simulink model "RoboBoat_NEDcallv12"  (R2014a)
settings: Solver=FixedStepDiscrete  StartTime=0.0  StopTime=inf  FixedStep=.1  RelTol=1e-3
undefined symbols (not defined in the file): Com1, Com2, Com3, Com4, DiscIntNeverNeededParam, standard
libraries: xpcseriallib x31, visiontextngfix x25, simulink x19, slrtlib x9, speedgoatlib_IO102 x3, speedgoatlib x1
(part 4 of 4)

== matlab function RoboBoat_NEDcallv12/Main FSM/Obstacle Navigation1/Exit Gate/Gate 1 (Red & White)/MATLAB Function ==
  data: Prob input; RPM output; ColorID input; Dist input; Ang input; CurrentHeading input; GPSLat input; GPSLong input; Timer input; DesiredHeading output; gateGPS output
function [RPM,DesiredHeading,gateGPS] = navigation(Prob,ColorID,Dist,Ang,CurrentHeading,GPSLat,GPSLong,Timer)

% Function performs one buoy navigation through the start speed gates. If
% no buoys are found by the LIDAR/Vision assembly then an incremented
% turning algorithm is executed to turn by 10 degrees per increment up to 
% 90 degrees either way of the inital heading

% Written by Edward Zhu

persistent LockHeading TimeLastFound Counter Turn TurnInc gateLat gateLong

if isempty(LockHeading) && isempty(TimeLastFound) && isempty(Counter) && isempty(Turn) && isempty(TurnInc)
    LockHeading = CurrentHeading;
    TimeLastFound = 0;
    Counter = 0;
    TurnInc = 30;
    Turn = TurnInc;
    gateLat = 0;
    gateLong = 0;
end

Distance = Dist/100;

BoatWidth = 0.75;
Buffer = atan(2*BoatWidth/Distance);

RedOffset = Ang + Buffer;
WhiteOffset = Ang - Buffer;

R = 6378137;

CurLat = (floor(GPSLat/100)+mod(GPSLat,100)/60)*pi/180;
CurLong = (ceil(GPSLong/100)-mod(-GPSLong,100)/60)*pi/180;

gateHeading = (mod(CurrentHeading + Ang, 360))*pi/180;

if ColorID == 1 && Prob > 0.9
    if Ang < 0
        DesiredHeading = mod(CurrentHeading - RedOffset, 360);
    else
        DesiredHeading = mod(CurrentHeading + RedOffset, 360);
    end
    RPM = 4000;
    GateFound = 1;
    TimeLastFound = Timer;
    gateLat =  asin(sin(CurLat)*cos(Distance/R) + cos(CurLat)*sin(Distance/R)*cos(gateHeading))*180/pi;
    gateLong = (CurLong + atan2(sin(gateHeading)*sin(Distance/R)*cos(CurLat),cos(Distance/R)-sin(CurLat)*sin(gateLat)))*180/pi;
elseif ColorID == 2 && Prob > 0.9
    DesiredHeading = mod(LockHeading - Turn, 360);
    RPM = 0;
    GateFound = 1;
    TimeLastFound = Timer;
%     DesiredHeading = mod(CurrentHeading - WhiteOffset, 360);
%     RPM = 4000;
%     GateFound = 1;
%     TimeLastFound = Timer;
%     gateLat =  asin(sin(CurLat)*cos(Distance/R) + cos(CurLat)*sin(Distance/R)*cos(gateHeading))*180/pi;
%     gateLong = (CurLong + atan2(sin(gateHeading)*sin(Distance/R)*cos(CurLat),cos(Distance/R)-sin(CurLat)*sin(gateLat)))*180/pi;
else
    DesiredHeading = CurrentHeading;
    RPM = 0;
    GateFound = 0;
end

gateGPS = [gateLat gateLong];
TimeNoBuoys = Timer - TimeLastFound;

if GateFound == 0 && TimeNoBuoys > 15
    RPM = 0;
    DesiredHeading = mod(LockHeading - Turn, 360);
    HeadingDiff = DesiredHeading - CurrentHeading;
    gateGPS = [gateLat gateLong];
    
    if HeadingDiff > 180
        HeadingDiff = HeadingDiff - 360;
    elseif HeadingDiff < -180
        HeadingDiff = HeadingDiff + 360;
    end
    
    if HeadingDiff < 3
        Counter = Counter + 1;
    else
        Counter = 0;
    end
    
    if Counter >= 15
        Turn = Turn + TurnInc;
        Counter = 0;
        if abs(Turn) > 90
            TurnInc = -TurnInc;
        end
    end
end

== matlab function RoboBoat_NEDcallv12/Main FSM/Obstacle Navigation1/Exit Gate/Gate 2 (White & White)/Distance ==
  data: Distance output; DesiredGPS input; GPSLat input; GPSLong input
function Distance  = DistCalc(DesiredGPS, GPSLat, GPSLong)

%Written by Anderson Lebbad on July 22, 2013
%Last Edited:

%Orients the boat towards a target GPS point before approaching it.
%This is done to keep the approach angle minimal, so the approach
%algorithm does not circle the target and never reach it.

%Parse input GPS and convert angles to radians
CurLat = (floor(GPSLat/100)+mod(GPSLat,100)/60)*pi/180;
CurLong = (floor(GPSLong/100)+mod(GPSLong,100)/60)*pi/180;
DesLat = (floor(DesiredGPS(1)/100)+mod(DesiredGPS(1),100)/60)*pi/180;
DesLong = (floor(DesiredGPS(2)/100)+mod(DesiredGPS(2),100)/60)*pi/180;
%Difference between lats and longs
DiffLat = DesLat - CurLat;
MidLat = cos((CurLat + DesLat)/2);
DiffLong = DesLong - CurLong;
%Radius of the earth in meters
R = 6378137;

%Calculate distance using the great-circle distance formula
%Formula documented here:
%   http://www.movable-type.co.uk/scripts/latlong.html
% a = sin(DiffLat/2)^2+sin(DiffLong/2)^2*cos(CurLat)*cos(DesLat);
% c = 2*atan2(sqrt(a), sqrt(1-a));
% Distance = R*c;

%Calculating distance using Pythagora's
a = DiffLong*MidLat;
b = DiffLat;
Distance = R*sqrt(a^2+b^2);

== matlab function RoboBoat_NEDcallv12/Sensors/Baseboard Serial/GPS Decode/LLA to NED ==
  data: GPSLat input; GPSLong input; Lat output; Long output
function [Lat, Long] = LLA2NEDfun(GPSLat,GPSLong)
%Written by Anderson Lebbad on September 20, 2014
%Last edited by:
%
%This function converts the NMEA formatted GPS values to degrees for
%latitude and longitude.

Lat = (floor(GPSLat/100)+mod(GPSLat,100)/60);
%Negative added for being in western hemisphere
Long = -(ceil(GPSLong/100)-mod(-GPSLong,100)/60);

end

== matlab function RoboBoat_NEDcallv12/Main FSM/Obstacle Navigation1/Exit Gate/Gate 2 (White & White)/MATLAB Function ==
  data: Prob input; RPM output; ColorID input; Dist input; Ang input; CurrentHeading input; GPSLat input; GPSLong input; Timer input; DesiredHeading output; gateGPS output
function [RPM,DesiredHeading,gateGPS] = navigation(Prob,ColorID,Dist,Ang,CurrentHeading,GPSLat,GPSLong,Timer)

% Function performs one buoy navigation through the start speed gates. If
% no buoys are found by the LIDAR/Vision assembly then an incremented
% turning algorithm is executed to turn by 10 degrees per increment up to 
% 90 degrees either way of the inital heading

% Written by Edward Zhu


persistent LockHeading TimeLastFound Counter Turn TurnInc gateLat gateLong

if isempty(LockHeading) && isempty(TimeLastFound) && isempty(Counter) && isempty(Turn) && isempty(TurnInc)
    LockHeading = CurrentHeading;
    TimeLastFound = 0;
    Counter = 0;
    TurnInc = 30;
    Turn = TurnInc;
    gateLat = 0;
    gateLong = 0;
end
Distance = Dist/100;
BoatWidth = 0.75;
Buffer = atan(2*BoatWidth/Distance);

RedOffset = Ang + Buffer;
WhiteOffset = Ang - Buffer;

R = 6378137;

CurLat = (floor(GPSLat/100)+mod(GPSLat,100)/60)*pi/180;
CurLong = (ceil(GPSLong/100)-mod(-GPSLong,100)/60)*pi/180;

gateHeading = (mod(CurrentHeading - Ang, 360))*pi/180;

if ColorID == 1 && Prob > 0.9
    DesiredHeading = mod(CurrentHeading - RedOffset, 360);
    RPM = 2000;
    GateFound = 1;
    TimeLastFound = Timer;
    gateLat =  asin(sin(CurLat)*cos(Distance/R) + cos(CurLat)*sin(Distance/R)*cos(gateHeading))*180/pi;
    gateLong = (CurLong + atan2(sin(gateHeading)*sin(Distance/R)*cos(CurLat),cos(Distance/R)-sin(CurLat)*sin(gateLat)))*180/pi;
elseif ColorID == 2 && Prob > 0.9
    DesiredHeading = mod(CurrentHeading - WhiteOffset, 360);
    RPM = 2000;
    GateFound = 1;
    TimeLastFound = Timer;
    gateLat =  asin(sin(CurLat)*cos(Distance/R) + cos(CurLat)*sin(Distance/R)*cos(gateHeading))*180/pi;
    gateLong = (CurLong + atan2(sin(gateHeading)*sin(Distance/R)*cos(CurLat),cos(Distance/R)-sin(CurLat)*sin(gateLat)))*180/pi;
else
    DesiredHeading = CurrentHeading;
    RPM = 0;
    GateFound = 0;
end

gateGPS = [gateLat gateLong];
TimeNoBuoys = Timer - TimeLastFound;

if GateFound == 0 && TimeNoBuoys > 15
    RPM = 0;
    DesiredHeading = mod(LockHeading - Turn, 360);
    HeadingDiff = DesiredHeading - CurrentHeading;
    gateGPS = [gateLat gateLong];
    
    if HeadingDiff > 180
        HeadingDiff = HeadingDiff - 360;
    elseif HeadingDiff < -180
        HeadingDiff = HeadingDiff + 360;
    end
    
    if HeadingDiff < 3
        Counter = Counter + 1;
    else
        Counter = 0;
    end
    
    if Counter >= 15
        Turn = Turn + TurnInc;
        Counter = 0;
        if abs(Turn) > 90
            TurnInc = -TurnInc;
        end
    end
end

== matlab function RoboBoat_NEDcallv12/Main FSM/Obstacle Navigation1/Exit Gate/Gate 3 (White & Green)/Distance ==
  data: Distance output; DesiredGPS input; GPSLat input; GPSLong input
function Distance  = DistCalc(DesiredGPS, GPSLat, GPSLong)

%Written by Anderson Lebbad on July 22, 2013
%Last Edited:

%Orients the boat towards a target GPS point before approaching it.
%This is done to keep the approach angle minimal, so the approach
%algorithm does not circle the target and never reach it.

%Parse input GPS and convert angles to radians
CurLat = (floor(GPSLat/100)+mod(GPSLat,100)/60)*pi/180;
CurLong = (floor(GPSLong/100)+mod(GPSLong,100)/60)*pi/180;
DesLat = (floor(DesiredGPS(1)/100)+mod(DesiredGPS(1),100)/60)*pi/180;
DesLong = (floor(DesiredGPS(2)/100)+mod(DesiredGPS(2),100)/60)*pi/180;
%Difference between lats and longs
DiffLat = DesLat - CurLat;
MidLat = cos((CurLat + DesLat)/2);
DiffLong = DesLong - CurLong;
%Radius of the earth in meters
R = 6378137;

%Calculate distance using the great-circle distance formula
%Formula documented here:
%   http://www.movable-type.co.uk/scripts/latlong.html
% a = sin(DiffLat/2)^2+sin(DiffLong/2)^2*cos(CurLat)*cos(DesLat);
% c = 2*atan2(sqrt(a), sqrt(1-a));
% Distance = R*c;

%Calculating distance using Pythagora's
a = DiffLong*MidLat;
b = DiffLat;
Distance = R*sqrt(a^2+b^2);

== matlab function RoboBoat_NEDcallv12/Main FSM/Obstacle Navigation1/Exit Gate/Gate 3 (White & Green)/MATLAB Function ==
  data: Prob input; RPM output; ColorID input; Dist input; Ang input; CurrentHeading input; GPSLat input; GPSLong input; Timer input; DesiredHeading output; gateGPS output
function [RPM,DesiredHeading,gateGPS] = navigation(Prob,ColorID,Dist,Ang,CurrentHeading,GPSLat,GPSLong,Timer)

% Function performs one buoy navigation through the start speed gates. If
% no buoys are found by the LIDAR/Vision assembly then an incremented
% turning algorithm is executed to turn by 10 degrees per increment up to 
% 90 degrees either way of the inital heading

% Written by Edward Zhu


persistent LockHeading TimeLastFound Counter Turn TurnInc gateLat gateLong

if isempty(LockHeading) && isempty(TimeLastFound) && isempty(Counter) && isempty(Turn) && isempty(TurnInc)
    LockHeading = CurrentHeading;
    TimeLastFound = 0;
    Counter = 0;
    TurnInc = 30;
    Turn = TurnInc;
    gateLat = 0;
    gateLong = 0;
end
Distance = Dist/100;
BoatWidth = 0.75;
Buffer = atan(2*BoatWidth/Distance);

WhiteOffset = Ang + Buffer;
GreenOffset = Ang - Buffer;

R = 6378137;

CurLat = (floor(GPSLat/100)+mod(GPSLat,100)/60)*pi/180;
CurLong = (ceil(GPSLong/100)-mod(-GPSLong,100)/60)*pi/180;

gateHeading = (mod(CurrentHeading - Ang, 360))*pi/180;

if ColorID == 2 && Prob > 0.9
    DesiredHeading = mod(LockHeading - Turn, 360);
    RPM = 0;
    GateFound = 1;
    TimeLastFound = Timer;
elseif ColorID == 3 && Prob > 0.9
    if Ang > 0
        DesiredHeading = mod(CurrentHeading - GreenOffset, 360);
    else
        DesiredHeading = mod(CurrentHeading + GreenOffset, 360);
    end
    RPM = 4000;
    GateFound = 1;
    TimeLastFound = Timer;
    gateLat =  asin(sin(CurLat)*cos(Distance/R) + cos(CurLat)*sin(Distance/R)*cos(gateHeading))*180/pi;
    gateLong = (CurLong + atan2(sin(gateHeading)*sin(Distance/R)*cos(CurLat),cos(Distance/R)-sin(CurLat)*sin(gateLat)))*180/pi;
else
    DesiredHeading = CurrentHeading;
    RPM = 0;
    GateFound = 0;
end

gateGPS = [gateLat gateLong];
TimeNoBuoys = Timer - TimeLastFound;

if GateFound == 0 && TimeNoBuoys > 15
    RPM = 0;
    DesiredHeading = mod(LockHeading - Turn, 360);
    HeadingDiff = DesiredHeading - CurrentHeading;
    gateGPS = [gateLat gateLong];
    
    if HeadingDiff > 180
        HeadingDiff = HeadingDiff - 360;
    elseif HeadingDiff < -180
        HeadingDiff = HeadingDiff + 360;
    end
    
    if HeadingDiff < 3
        Counter = Counter + 1;
    else
        Counter = 0;
    end
    
    if Counter >= 15
        Turn = Turn + TurnInc;
        Counter = 0;
        if abs(Turn) > 90
            TurnInc = -TurnInc;
        end
    end
end

== matlab function RoboBoat_NEDcallv12/Main FSM/Obstacle Navigation1/Exit Gate/MATLAB Function ==
  data: gateID input; outputSelector output; gate1En output; gate2En output; gate3En output
function [outputSelector,gate1En,gate2En,gate3En] = gateSelector(gateID)
% Determines which colors to filter for based on the gateID as received
% from the judges

gate1En = 0;
gate2En = 0;
gate3En = 0;

if gateID == 1
    gate1En = 1;
    outputSelector = 1;
elseif gateID == 2
    gate2En = 1;
    outputSelector = 2;
else
    gate3En = 1;
    outputSelector = 3;
end

== matlab function RoboBoat_NEDcallv12/Sinks/actuators/analog output/Subsystem/Heading Controller/MATLAB Function ==
  data: HeadingDesired input; steering output; CompassHeading input
function steering = CalcSteering(HeadingDesired, CompassHeading)

%Written by Anderson Lebbad on May 29, 2015
%Last Edited: Anderson Lebbad on June 7, 2015
%   Simplified using mod division

%Calculates the difference between the desired and current heading to be
%used for steering

steering = HeadingDesired - CompassHeading;
%atan2 in radians, input and output in degrees
steering = atan2(sin(steering*pi/180),cos(steering*pi/180))*180/pi;

== matlab function RoboBoat_NEDcallv12/Main FSM/Obstacle Navigation1/Enter Gate/Gate 1 (Red & White)/Distance ==
  data: Distance output; DesiredGPS input; GPSLat input; GPSLong input
function Distance  = DistCalc(DesiredGPS, GPSLat, GPSLong)

%Written by Anderson Lebbad on July 22, 2013
%Last Edited:

%Orients the boat towards a target GPS point before approaching it.
%This is done to keep the approach angle minimal, so the approach
%algorithm does not circle the target and never reach it.

%Parse input GPS and convert angles to radians
CurLat = (floor(GPSLat/100)+mod(GPSLat,100)/60)*pi/180;
CurLong = (floor(GPSLong/100)+mod(GPSLong,100)/60)*pi/180;
DesLat = (floor(DesiredGPS(1)/100)+mod(DesiredGPS(1),100)/60)*pi/180;
DesLong = (floor(DesiredGPS(2)/100)+mod(DesiredGPS(2),100)/60)*pi/180;
%Difference between lats and longs
DiffLat = DesLat - CurLat;
MidLat = cos((CurLat + DesLat)/2);
DiffLong = DesLong - CurLong;
%Radius of the earth in meters
R = 6378137;

%Calculate distance using the great-circle distance formula
%Formula documented here:
%   http://www.movable-type.co.uk/scripts/latlong.html
% a = sin(DiffLat/2)^2+sin(DiffLong/2)^2*cos(CurLat)*cos(DesLat);
% c = 2*atan2(sqrt(a), sqrt(1-a));
% Distance = R*c;

%Calculating distance using Pythagora's
a = DiffLong*MidLat;
b = DiffLat;
Distance = R*sqrt(a^2+b^2);

== matlab function RoboBoat_NEDcallv12/Main FSM/Obstacle Navigation1/Enter Gate/Gate 1 (Red & White)/MATLAB Function ==
  data: Prob input; RPM output; ColorID input; Dist input; Ang input; CurrentHeading input; GPSLat input; GPSLong input; Timer input; DesiredHeading output; gateGPS output
function [RPM,DesiredHeading,gateGPS] = navigation(Prob,ColorID,Dist,Ang,CurrentHeading,GPSLat,GPSLong,Timer)

% Function performs one buoy navigation through the start speed gates. If
% no buoys are found by the LIDAR/Vision assembly then an incremented
% turning algorithm is executed to turn by 10 degrees per increment up to 
% 90 degrees either way of the inital heading

% Written by Edward Zhu

persistent LockHeading TimeLastFound Counter Turn TurnInc gateLat gateLong

if isempty(LockHeading) && isempty(TimeLastFound) && isempty(Counter) && isempty(Turn) && isempty(TurnInc)
    LockHeading = CurrentHeading;
    TimeLastFound = 0;
    Counter = 0;
    TurnInc = 30;
    Turn = TurnInc;
    gateLat = 0;
    gateLong = 0;
end

Distance = Dist/100;

BoatWidth = 0.75;
Buffer = atan(2*BoatWidth/Distance);

RedOffset = Ang + Buffer;
WhiteOffset = Ang - Buffer;

R = 6378137;

CurLat = (floor(GPSLat/100)+mod(GPSLat,100)/60)*pi/180;
CurLong = (ceil(GPSLong/100)-mod(-GPSLong,100)/60)*pi/180;

gateHeading = (mod(CurrentHeading + Ang, 360))*pi/180;

if ColorID == 1 && Prob > 0.9
    if Ang < 0
        DesiredHeading = mod(CurrentHeading - RedOffset, 360);
    else
        DesiredHeading = mod(CurrentHeading + RedOffset, 360);
    end
    RPM = 4000;
    GateFound = 1;
    TimeLastFound = Timer;
    gateLat =  asin(sin(CurLat)*cos(Distance/R) + cos(CurLat)*sin(Distance/R)*cos(gateHeading))*180/pi;
    gateLong = (CurLong + atan2(sin(gateHeading)*sin(Distance/R)*cos(CurLat),cos(Distance/R)-sin(CurLat)*sin(gateLat)))*180/pi;
elseif ColorID == 2 && Prob > 0.9
    DesiredHeading = mod(LockHeading - Turn, 360);
    RPM = 0;
    GateFound = 1;
    TimeLastFound = Timer;
%     DesiredHeading = mod(CurrentHeading - WhiteOffset, 360);
%     RPM = 4000;
%     GateFound = 1;
%     TimeLastFound = Timer;
%     gateLat =  asin(sin(CurLat)*cos(Distance/R) + cos(CurLat)*sin(Distance/R)*cos(gateHeading))*180/pi;
%     gateLong = (CurLong + atan2(sin(gateHeading)*sin(Distance/R)*cos(CurLat),cos(Distance/R)-sin(CurLat)*sin(gateLat)))*180/pi;
else
    DesiredHeading = CurrentHeading;
    RPM = 0;
    GateFound = 0;
end

gateGPS = [gateLat gateLong];
TimeNoBuoys = Timer - TimeLastFound;

if GateFound == 0 && TimeNoBuoys > 15
    RPM = 0;
    DesiredHeading = mod(LockHeading - Turn, 360);
    HeadingDiff = DesiredHeading - CurrentHeading;
    gateGPS = [gateLat gateLong];
    
    if HeadingDiff > 180
        HeadingDiff = HeadingDiff - 360;
    elseif HeadingDiff < -180
        HeadingDiff = HeadingDiff + 360;
    end
    
    if HeadingDiff < 3
        Counter = Counter + 1;
    else
        Counter = 0;
    end
    
    if Counter >= 15
        Turn = Turn + TurnInc;
        Counter = 0;
        if abs(Turn) > 90
            TurnInc = -TurnInc;
        end
    end
end

== matlab function RoboBoat_NEDcallv12/Main FSM/Obstacle Navigation1/Enter Gate/Gate 2 (White & White)/Distance ==
  data: Distance output; DesiredGPS input; GPSLat input; GPSLong input
function Distance  = DistCalc(DesiredGPS, GPSLat, GPSLong)

%Written by Anderson Lebbad on July 22, 2013
%Last Edited:

%Orients the boat towards a target GPS point before approaching it.
%This is done to keep the approach angle minimal, so the approach
%algorithm does not circle the target and never reach it.

%Parse input GPS and convert angles to radians
CurLat = (floor(GPSLat/100)+mod(GPSLat,100)/60)*pi/180;
CurLong = (floor(GPSLong/100)+mod(GPSLong,100)/60)*pi/180;
DesLat = (floor(DesiredGPS(1)/100)+mod(DesiredGPS(1),100)/60)*pi/180;
DesLong = (floor(DesiredGPS(2)/100)+mod(DesiredGPS(2),100)/60)*pi/180;
%Difference between lats and longs
DiffLat = DesLat - CurLat;
MidLat = cos((CurLat + DesLat)/2);
DiffLong = DesLong - CurLong;
%Radius of the earth in meters
R = 6378137;

%Calculate distance using the great-circle distance formula
%Formula documented here:
%   http://www.movable-type.co.uk/scripts/latlong.html
% a = sin(DiffLat/2)^2+sin(DiffLong/2)^2*cos(CurLat)*cos(DesLat);
% c = 2*atan2(sqrt(a), sqrt(1-a));
% Distance = R*c;

%Calculating distance using Pythagora's
a = DiffLong*MidLat;
b = DiffLat;
Distance = R*sqrt(a^2+b^2);

== matlab function RoboBoat_NEDcallv12/Main FSM/Obstacle Navigation1/Enter Gate/Gate 2 (White & White)/MATLAB Function ==
  data: Prob input; RPM output; ColorID input; Dist input; Ang input; CurrentHeading input; GPSLat input; GPSLong input; Timer input; DesiredHeading output; gateGPS output
function [RPM,DesiredHeading,gateGPS] = navigation(Prob,ColorID,Dist,Ang,CurrentHeading,GPSLat,GPSLong,Timer)

% Function performs one buoy navigation through the start speed gates. If
% no buoys are found by the LIDAR/Vision assembly then an incremented
% turning algorithm is executed to turn by 10 degrees per increment up to 
% 90 degrees either way of the inital heading

% Written by Edward Zhu


persistent LockHeading TimeLastFound Counter Turn TurnInc gateLat gateLong

if isempty(LockHeading) && isempty(TimeLastFound) && isempty(Counter) && isempty(Turn) && isempty(TurnInc)
    LockHeading = CurrentHeading;
    TimeLastFound = 0;
    Counter = 0;
    TurnInc = 30;
    Turn = TurnInc;
    gateLat = 0;
    gateLong = 0;
end
Distance = Dist/100;
BoatWidth = 0.75;
Buffer = atan(2*BoatWidth/Distance);

RedOffset = Ang + Buffer;
WhiteOffset = Ang - Buffer;

R = 6378137;

CurLat = (floor(GPSLat/100)+mod(GPSLat,100)/60)*pi/180;
CurLong = (ceil(GPSLong/100)-mod(-GPSLong,100)/60)*pi/180;

gateHeading = (mod(CurrentHeading - Ang, 360))*pi/180;

if ColorID == 1 && Prob > 0.9
    DesiredHeading = mod(CurrentHeading - RedOffset, 360);
    RPM = 2000;
    GateFound = 1;
    TimeLastFound = Timer;
    gateLat =  asin(sin(CurLat)*cos(Distance/R) + cos(CurLat)*sin(Distance/R)*cos(gateHeading))*180/pi;
    gateLong = (CurLong + atan2(sin(gateHeading)*sin(Distance/R)*cos(CurLat),cos(Distance/R)-sin(CurLat)*sin(gateLat)))*180/pi;
elseif ColorID == 2 && Prob > 0.9
    DesiredHeading = mod(CurrentHeading - WhiteOffset, 360);
    RPM = 2000;
    GateFound = 1;
    TimeLastFound = Timer;
    gateLat =  asin(sin(CurLat)*cos(Distance/R) + cos(CurLat)*sin(Distance/R)*cos(gateHeading))*180/pi;
    gateLong = (CurLong + atan2(sin(gateHeading)*sin(Distance/R)*cos(CurLat),cos(Distance/R)-sin(CurLat)*sin(gateLat)))*180/pi;
else
    DesiredHeading = CurrentHeading;
    RPM = 0;
    GateFound = 0;
end

gateGPS = [gateLat gateLong];
TimeNoBuoys = Timer - TimeLastFound;

if GateFound == 0 && TimeNoBuoys > 15
    RPM = 0;
    DesiredHeading = mod(LockHeading - Turn, 360);
    HeadingDiff = DesiredHeading - CurrentHeading;
    gateGPS = [gateLat gateLong];
    
    if HeadingDiff > 180
        HeadingDiff = HeadingDiff - 360;
    elseif HeadingDiff < -180
        HeadingDiff = HeadingDiff + 360;
    end
    
    if HeadingDiff < 3
        Counter = Counter + 1;
    else
        Counter = 0;
    end
    
    if Counter >= 15
        Turn = Turn + TurnInc;
        Counter = 0;
        if abs(Turn) > 90
            TurnInc = -TurnInc;
        end
    end
end

== matlab function RoboBoat_NEDcallv12/Main FSM/Obstacle Navigation1/Enter Gate/Gate 3 (White & Green)/Distance ==
  data: Distance output; DesiredGPS input; GPSLat input; GPSLong input
function Distance  = DistCalc(DesiredGPS, GPSLat, GPSLong)

%Written by Anderson Lebbad on July 22, 2013
%Last Edited:

%Orients the boat towards a target GPS point before approaching it.
%This is done to keep the approach angle minimal, so the approach
%algorithm does not circle the target and never reach it.

%Parse input GPS and convert angles to radians
CurLat = (floor(GPSLat/100)+mod(GPSLat,100)/60)*pi/180;
CurLong = (floor(GPSLong/100)+mod(GPSLong,100)/60)*pi/180;
DesLat = (floor(DesiredGPS(1)/100)+mod(DesiredGPS(1),100)/60)*pi/180;
DesLong = (floor(DesiredGPS(2)/100)+mod(DesiredGPS(2),100)/60)*pi/180;
%Difference between lats and longs
DiffLat = DesLat - CurLat;
MidLat = cos((CurLat + DesLat)/2);
DiffLong = DesLong - CurLong;
%Radius of the earth in meters
R = 6378137;

%Calculate distance using the great-circle distance formula
%Formula documented here:
%   http://www.movable-type.co.uk/scripts/latlong.html
% a = sin(DiffLat/2)^2+sin(DiffLong/2)^2*cos(CurLat)*cos(DesLat);
% c = 2*atan2(sqrt(a), sqrt(1-a));
% Distance = R*c;

%Calculating distance using Pythagora's
a = DiffLong*MidLat;
b = DiffLat;
Distance = R*sqrt(a^2+b^2);

== matlab function RoboBoat_NEDcallv12/Main FSM/Obstacle Navigation1/Obstacle Navigation/GPS: Bee Line/Orient/Desired Heading ==
  data: DesiredGPS input; DesiredHeading output; GPSLat input; GPSLong input
function DesiredHeading = Orient(DesiredGPS, GPSLat, GPSLong)

%Written by Anderson Lebbad on July 22, 2013
%Last Edited: Edward Zhu on July 5, 2014

% Edit:
% Changed calculation to use positive lat and negative long

%Orients the boat towards a target GPS point before approaching it.
%This is done to keep the approach angle minimal, so the approach
%algorithm does not circle the target and never reach it.

%Parse input GPS and convert angles to radians
CurLat = (floor(GPSLat/100)+mod(GPSLat,100)/60)*pi/180;
CurLong = (ceil(GPSLong/100)-mod(-GPSLong,100)/60)*pi/180;
DesLat = (floor(DesiredGPS(1)/100)+mod(DesiredGPS(1),100)/60)*pi/180;
DesLong = (ceil(DesiredGPS(2)/100)-mod(-DesiredGPS(2),100)/60)*pi/180;

%Difference between longs
DiffLong = DesLong - CurLong;

%Calculate initial bearing - formula documented here: 
%   http://www.movable-type.co.uk/scripts/latlong.html
y = sin(DiffLong)*cos(DesLat);
x = cos(CurLat)*sin(DesLat)-sin(CurLat)*cos(DesLat)*cos(DiffLong);
DesiredHeading = mod(atan2(y, x)*180/pi + 360, 360);

== matlab function RoboBoat_NEDcallv12/Main FSM/Obstacle Navigation1/GPS: Center/Approach/MATLAB Function ==
  data: GPSLat input; out output; GPSLong input; IMULat input; IMULong input
function out = dataFormat(GPSLat, GPSLong, IMULat, IMULong)
%#codegen
out = [GPSLat GPSLong IMULat IMULong];

== matlab function RoboBoat_NEDcallv12/Main FSM/Obstacle Navigation1/GPS: Center/GPS Enabler ==
  data: Finished input; GPSMode output; OrientEnable output; ApproachEnable output
function [GPSMode, OrientEnable, ApproachEnable] =...
    GPSEnable(Finished)

%Written by Anderson Lebbad on July 22, 2013
%Last Edited: July 27, 2013
%   Removed Termination Block

%This function enables GPS tasks. First the boat orients towards the
%target, then it approaches it.


%Parse Finished signal
OrientFinished = Finished(1);


%Initialize Enablers
OrientEnable = 0;
ApproachEnable = 0;


%Switches the enable signal based on which task is flagged as done.
if OrientFinished == 0
    OrientEnable = 1;
    GPSMode = 1;
else
    ApproachEnable = 1;
    GPSMode = 2;
end

== matlab function RoboBoat_NEDcallv12/Main FSM/Obstacle Navigation1/GPS: Center/Orient/Within Range ==
  data: DesiredHeading input; Finished output; Compass input
function Finished = OrientLocked(DesiredHeading, Compass)

%Written by Anderson Lebbad on July 22, 2013
%Last Edited:

%This function checks to see if the target heading has been reached and 
%sends a finished signal when it has.

HeadingDiff = DesiredHeading - Compass;

%Sets the range for the difference angle to be -180 to +180
if HeadingDiff > 180
    HeadingDiff = HeadingDiff - 360;
elseif HeadingDiff < -180
    HeadingDiff = HeadingDiff + 360;
end

%If the Heading is within 3 degrees, the angle is close enough to send a
%finished signal
if abs(HeadingDiff) < 3
    Finished = 1;
else
    Finished = 0;
end

== matlab function RoboBoat_NEDcallv12/Main FSM/Obstacle Navigation1/Obstacle Navigation/Dodge/Nav Logic ==
  data: CurrentHeading input; Dist input; Ang input; ObstDist output; RPM output; DesiredHeading output; Timer input; Timeout input; DodgeIncomplete output
 function [ObstDist, RPM, DesiredHeading, DodgeIncomplete] = NavLogic(CurrentHeading,...
    Dist, Ang, Timer, Timeout)

%Written by Anderson Lebbad on August 20, 2013
%Last Edited by:

%Determines the signals for driving through the buoy channel based on the
%bounding box and centroid signals from both the red and green detection
%blocks.

persistent TimeLastFound heldHeading

ObstDist = Dist / 100;

if isempty(TimeLastFound) && isempty(heldHeading)
    TimeLastFound = 0;
    heldHeading = CurrentHeading;
end

if ObstDist > 0 && ObstDist <= 2
    %Buffer for single buoy offset is the angle to twice the boat's width off of the
    %center of the buoy
    BoatWidth = .75;
    Buffer = atan(2 * BoatWidth / ObstDist) * 180 / pi;
    
    if Ang < 0
        ObstOffset = Ang + Buffer;
    else
        ObstOffset = Ang - Buffer;
    end
    
    DesiredHeading = mod(CurrentHeading + ObstOffset, 360);
    RPM = 2800;
    
    TimeLastFound = Timer;
    heldHeading = CurrentHeading;
    
    DodgeIncomplete = 1;
    
else
    DesiredHeading = heldHeading;
    RPM = 2800;
    
    if Timer-TimeLastFound < Timeout
        DodgeIncomplete = 1;
    else
        DodgeIncomplete = 0;
    end

end

== matlab function RoboBoat_NEDcallv12/Sensors/1020 Comms/Data Update1 ==
  data: Valid input; ControlMode input; V output; C output; L output; A output; Data input; D1 output; D2 output; D3 output; D4 output; D5 output; D6 output; D7 output; D8 output; D9 output; D10 output; D11 output; D12 output; D13 output; D14 output; D15 output; D16 output; D17 output; D18 output; D19 output; D20 output; D21 output; D22 output; D23 output; D24 output; Activate input
function [V,C,L,A,D1,D2,D3,D4,D5,D6,D7,D8,D9,D10,D11,D12,D13,D14,D15,D16,D17,...
    D18,D19,D20,D21,D22,D23,D24] = dataSplit(Valid,ControlMode,Data,Activate)
%Written by Anderson Lebbad on August 10, 2014
%Last Edited by: Anderson Lebbad on September 11, 2014

%This function splits the data vector into the twelve channels it is
%composed of for communication

persistent HoldData

A = Activate;

if isempty(HoldData)
    HoldData = zeros(26,1);
end

L = 8;

if Valid == 1
    HoldData(1) = Valid;
    HoldData(2) = ControlMode;
    HoldData(3) = Data(1);
    HoldData(4) = Data(2);
    HoldData(5) = Data(3);
    HoldData(6) = Data(4);
    HoldData(7) = Data(5);
    HoldData(8) = Data(6);
    HoldData(9) = Data(7);
    HoldData(10) = Data(8);
    HoldData(11) = Data(9);
    HoldData(12) = Data(10);
    HoldData(13) = Data(11);
    HoldData(14) = Data(12);
    HoldData(15) = Data(13);
    HoldData(16) = Data(14);
    HoldData(17) = Data(15);
    HoldData(18) = Data(16);
    HoldData(19) = Data(17);
    HoldData(20) = Data(18);
    HoldData(21) = Data(19);
    HoldData(22) = Data(20);
    HoldData(23) = Data(21);
    HoldData(24) = Data(22);
    HoldData(25) = Data(23);
    HoldData(26) = Data(24);
end

V = HoldData(1);
C = HoldData(2);
D1 = HoldData(3);
D2 = HoldData(4);
D3 = HoldData(5);
D4 = HoldData(6);
D5 = HoldData(7);
D6 = HoldData(8);
D7 = HoldData(9);
D8 = HoldData(10);
D9 = HoldData(11);
D10 = HoldData(12);
D11 = HoldData(13);
D12 = HoldData(14);
D13 = HoldData(15);
D14 = HoldData(16);
D15 = HoldData(17);
D16 = HoldData(18);
D17 = HoldData(19);
D18 = HoldData(20);
D19 = HoldData(21);
D20 = HoldData(22);
D21 = HoldData(23);
D22 = HoldData(24);
D23 = HoldData(25);
D24 = HoldData(26);

end

== matlab function RoboBoat_NEDcallv12/Sensors/1020 Comms/MATLAB Function2 ==
  data: Time input; asciiLIT output; Sequence input
% This function creates the light tower message to be sent from 
% Speedgoat in ascii code
% Written by: Edward Zhu
% Date: 9/17/14

function asciiLIT = asciiLITEncoder(Time, Sequence)

% Initialize output message vector as the serial output block expects 128
% character message
asciiLIT = uint8(zeros(1,128));

% Convert static strings to ascii code
asciiMsgID = uint8('$RXLIT,');
asciiComma = uint8(',');
asciiTeamID = uint8('FAUVU,');
asciiMsgEnd = uint8('*');
asciiMsgCRLF = [13 10];

% Convert UTC Time input (hhmmss) into ascii code
asciiTime = uint8(zeros(1,7));
asciiTime(7) = asciiComma;

for timeChar = 1:6
    asciiTime(timeChar) = floor(mod(Time,10^(7-timeChar))/...
        10^(6-timeChar)) + 48;
end

% Convert the light sequece into ascii code (1 = R, 2 = B, 3 = G)
asciiSeq = uint8(zeros(1,4)+32);
asciiSeq(4) = asciiMsgEnd;

if Sequence(1) > 0 && Sequence(2) > 0 && Sequence(3) > 0
    for seqChar = 1:3
        if Sequence(seqChar) == 1
            Sequence(seqChar) = uint8('R');
        elseif Sequence(seqChar) == 2
            Sequence(seqChar) = uint8('B');
        elseif Sequence(seqChar) == 3
            Sequence(seqChar) = uint8('G');
        end
    end
    asciiSeq(1:3) = Sequence;
end

% Concat individual ascii arrays into one array
asciiPreChkSum = cat(2,asciiMsgID,asciiTime,asciiTeamID,asciiSeq);

% Calculate the checksum of the message from the '$' to the '*' and convert
% to hex
chkSum = uint8(0);

for chksumChar = 1:(length(asciiPreChkSum)-2)
    chkSum = bitxor(chkSum,asciiPreChkSum(chksumChar+1));
end

% Convert the checksum to ascii
chkSum = dec2hex(chkSum);
asciiChkSum = uint8(zeros(1,length(chkSum))+32);
for i = 1:length(chkSum)
    asciiChkSum(i) = uint8(chkSum(i));
end

% Concat the checksum and the '/r/n' to the end of the message
asciiPostChkSum = cat(2,asciiPreChkSum,asciiChkSum,asciiMsgCRLF);

% Output the final message
asciiLIT(1:length(asciiPostChkSum)) = asciiPostChkSum;

== matlab function RoboBoat_NEDcallv12/Main FSM/Obstacle Navigation2/MATLAB Function ==
  data: requestNumOut output; CP input; requestNumIn input; Finished output
function [requestNumOut, Finished] = requestSender(CP, requestNumIn)

persistent counter
if isempty(counter)
    counter = 0;
end

if CP < 1
    requestNumOut = requestNumIn;
    Finished = 0;
else
    counter = counter + 1;
    if counter >= 50
        requestNumOut = 0;
        Finished = 1;
    else
        requestNumOut = requestNumIn;
        Finished = 0;
    end
end

== matlab function RoboBoat_NEDcallv12/Main FSM/Shotgun Speedgate/MATLAB Function ==
  data: Heading input; LockedHeading output
function LockedHeading = HeadingLock(Heading)

persistent lock

if isempty(lock)
    lock = Heading;
end

LockedHeading = lock;

== matlab function RoboBoat_NEDcallv12/Main FSM/Shotgun Speedgate/MATLAB Function1 ==
  data: desiredHeading input; out output; Heading input
function out = dataOrganizer(desiredHeading, Heading)
%#codegen

out = [desiredHeading Heading];
